simulink model "experiments2_cl"  (R2017a)
settings: Solver=VariableStepAuto  StartTime=0.0  StopTime=45  RelTol=1e-3
settings Model: Creator=Mr.li  LastModifiedBy=Mr.li

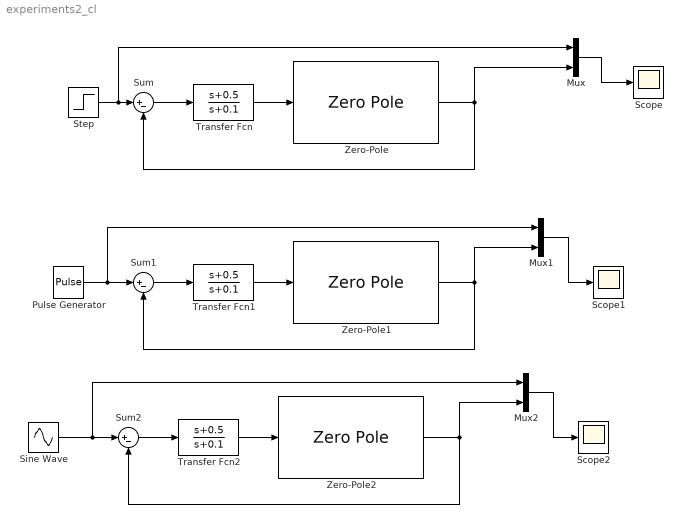
== system experiments2_cl ==
  Mux : Mux  Inputs=2
  Mux1 : Mux  Inputs=2
  Mux2 : Mux  Inputs=2
  Pulse Generator : DiscretePulseGenerator  PulseType=Time based  Period=15  PulseWidth=50
  Scope : Scope
  Scope1 : Scope
  Scope2 : Scope
  Sine Wave : Sin  Frequency=2*pi/15  SampleTime=0
  Step : Step  SampleTime=0
  Sum : Sum  Inputs=|+-
  Sum1 : Sum  Inputs=|+-
  Sum2 : Sum  Inputs=|+-
  Transfer Fcn : TransferFcn  Numerator=[1 0.5]  Denominator=[1 0.1]
  Transfer Fcn1 : TransferFcn  Numerator=[1 0.5]  Denominator=[1 0.1]
  Transfer Fcn2 : TransferFcn  Numerator=[1 0.5]  Denominator=[1 0.1]
  Zero-Pole : ZeroPole  Zeros=[]  Poles=[0 -2 -10]  Gain=20
  Zero-Pole1 : ZeroPole  Zeros=[]  Poles=[0 -2 -10]  Gain=20
  Zero-Pole2 : ZeroPole  Zeros=[]  Poles=[0 -2 -10]  Gain=20
  wires:
  Transfer Fcn/1 -> Zero-Pole/1
  Zero-Pole/1 -> Mux/2, Sum/2
  Step/1 -> Mux/1, Sum/1
  Sum/1 -> Transfer Fcn/1
  Sum1/1 -> Transfer Fcn1/1
  Zero-Pole1/1 -> Mux1/2, Sum1/2
  Transfer Fcn1/1 -> Zero-Pole1/1
  Pulse Generator/1 -> Mux1/1, Sum1/1
  Mux/1 -> Scope/1
  Mux1/1 -> Scope1/1
  Mux2/1 -> Scope2/1
  Sine Wave/1 -> Sum2/1, Mux2/1
  Transfer Fcn2/1 -> Zero-Pole2/1
  Zero-Pole2/1 -> Sum2/2, Mux2/2
  Sum2/1 -> Transfer Fcn2/1
